simulink model "line_following_robot_sim"  (R2024b)
settings: Solver=VariableStepAuto  StartTime=0.0  StopTime=10.0  RelTol=1e-3
settings Model: Creator=Timi Banjo  LastModifiedBy=Caleb
settings OptimizationCC: ReuseModelBlockBuffer=off
settings RTWCC: GPUComputeCapability=3.5

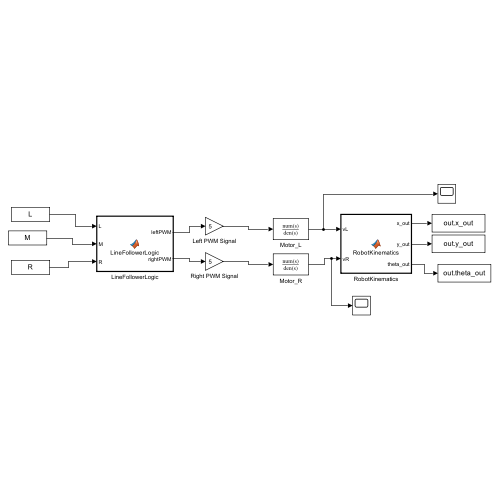
[thumbnail: Simulink's stored preview of the top-level diagram]
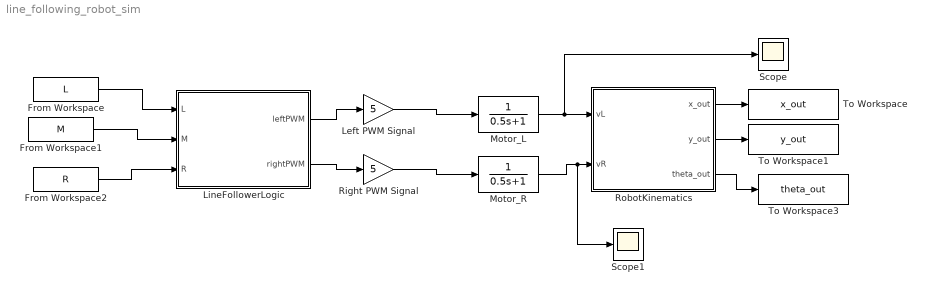
== system line_following_robot_sim ==
  From Workspace : FromWorkspace  VariableName=L
  From Workspace1 : FromWorkspace  VariableName=M
  From Workspace2 : FromWorkspace  VariableName=R
  Left PWM Signal : Gain  Gain=5
  LineFollowerLogic : MATLAB Function  TreatAsAtomicUnit=on
  Motor_L : TransferFcn  Denominator=[0.5 1]
  Motor_R : TransferFcn  Denominator=[0.5 1]
  Right PWM Signal : Gain  Gain=5
  RobotKinematics : MATLAB Function  TreatAsAtomicUnit=on
  Scope : Scope
  Scope1 : Scope
  To Workspace : ToWorkspace  VariableName=x_out  SaveFormat=Timeseries  SampleTime=-1
  To Workspace1 : ToWorkspace  VariableName=y_out  SaveFormat=Timeseries  SampleTime=-1
  To Workspace3 : ToWorkspace  VariableName=theta_out  SaveFormat=Timeseries  SampleTime=-1
  wires:
  From Workspace1/1 -> LineFollowerLogic/2(M)
  From Workspace/1 -> LineFollowerLogic/1(L)
  From Workspace2/1 -> LineFollowerLogic/3(R)
  LineFollowerLogic/2(rightPWM) -> Right PWM Signal/1
  LineFollowerLogic/1(leftPWM) -> Left PWM Signal/1
  Right PWM Signal/1 -> Motor_R/1
  Left PWM Signal/1 -> Motor_L/1
  Motor_L/1 -> Scope/1, RobotKinematics/1(vL)
  Motor_R/1 -> Scope1/1, RobotKinematics/2(vR)
  RobotKinematics/2(y_out) -> To Workspace1/1
  RobotKinematics/1(x_out) -> To Workspace/1
  RobotKinematics/3(theta_out) -> To Workspace3/1

== matlab function line_following_robot_sim/RobotKinematics ==
  settings: updateMethod=DISCRETE
  data: vL input; x_out output; vR input; y_out output; theta_out output
function [x_out, y_out, theta_out] = RobotKinematics(vL, vR)
% Simulates robot position over time using differential drive kinematics

% Constants
dt = 0.1;         % Simulation time step (seconds)
d = 0.2;          % Distance between wheels (meters)

% Persistent state variables
persistent x y theta
if isempty(x)
    x = 0;
    y = 0;
    theta = 0;
end

% Compute linear and angular velocity
v = (vL + vR) / 2;
omega = (vR - vL) / d;

% Update robot position and heading
x = x + v * cos(theta) * dt;
y = y + v * sin(theta) * dt;
theta = theta + omega * dt;

% Output updated values
x_out = x;
y_out = y;
theta_out = theta;
end

== matlab function line_following_robot_sim/LineFollowerLogic ==
  data: L input; leftPWM output; M input; R input; rightPWM output
function [leftPWM, rightPWM] = LineFollowerLogic(L, M, R)
    if M == 1 && L == 0 && R == 0
        leftPWM = 1; rightPWM = 1;     % Move forward
    elseif L == 1 && M == 1
        leftPWM = 0.5; rightPWM = 1;   % Soft left
    elseif R == 1 && M == 1
        leftPWM = 1; rightPWM = 0.5;   % Soft right
    elseif L == 1 && M == 0
        leftPWM = 0.3; rightPWM = 1;   % Hard left
    elseif R == 1 && M == 0
        leftPWM = 1; rightPWM = 0.3;   % Hard right
    else
        leftPWM = 0; rightPWM = 0;     % Stop
    end
end
